simulink model "IMP_SIMPLE"  (R2022a)
settings: Solver=VariableStepAuto  StartTime=0.0  StopTime=30  RelTol=1e-3
undefined symbols (not defined in the file): Ad, Ap, Bd, Bp, Cp, ka, ki
libraries: simulink x1
settings Model: Creator=Eduardo Toro Bernal  LastModifiedBy=Eduardo Toro Bernal

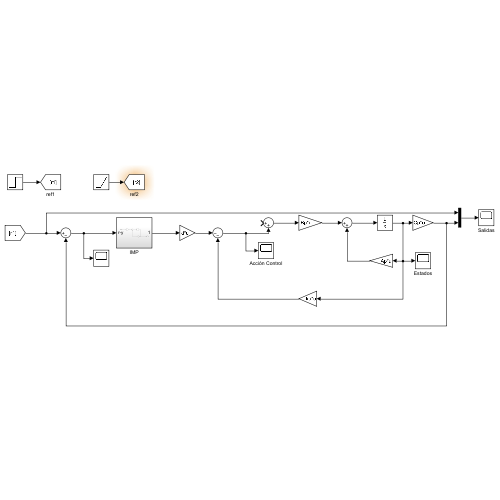
[thumbnail: Simulink's stored preview of the top-level diagram]
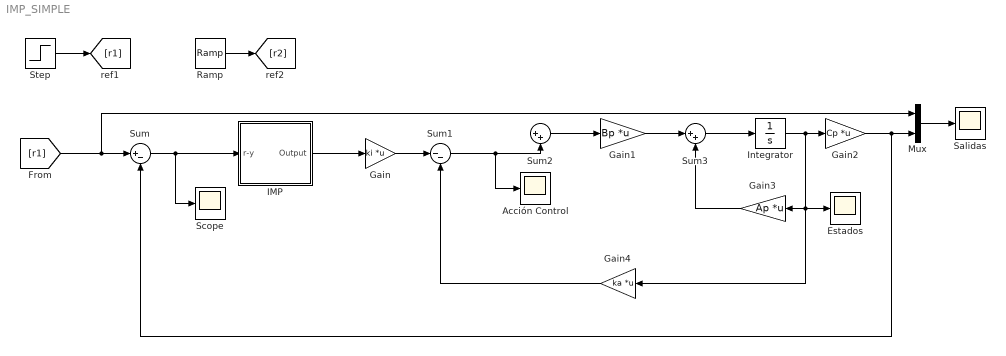
== system IMP_SIMPLE ==
  Acción Control : Scope
  Estados : Scope
  Gain : Gain  Gain=ki  Multiplication=Matrix(K*u)
  Gain1 : Gain  Gain=Bp  Multiplication=Matrix(K*u)
  Gain2 : Gain  Gain=Cp  Multiplication=Matrix(K*u)
  Gain3 : Gain  Gain=Ap  Multiplication=Matrix(K*u)
  Gain4 : Gain  Gain=ka  Multiplication=Matrix(K*u)
  IMP : Subsystem
  Integrator : Integrator
  Mux : Mux  Inputs=2
  Ramp : simulink/Sources/Ramp  slope=1  start=0  InitialOutput=0
  Salidas : Scope
  Scope : Scope
  Step : Step  SampleTime=0
  Sum : Sum  Inputs=|+-
  Sum1 : Sum  Inputs=|--
  Sum2 : Sum  Inputs=|++
  Sum3 : Sum  Inputs=|++
  wires:
  Sum/1 -> Scope/1, IMP/1(r-y)
  IMP/1(Output) -> Gain/1
  Gain/1 -> Sum1/1
  Sum1/1 -> Acción Control/1, Sum2/2
  Sum2/1 -> Gain1/1
  Gain1/1 -> Sum3/1
  Sum3/1 -> Integrator/1
  Integrator/1 -> Estados/1, Gain4/1, Gain3/1, Gain2/1
  Mux/1 -> Salidas/1
  Gain2/1 -> Sum/2, Mux/2
  [r1] -> Mux/1, Sum/1
  Gain3/1 -> Sum3/2
  Gain4/1 -> Sum1/2
  Step/1 -> [r1]
  Ramp/1 -> [r2]

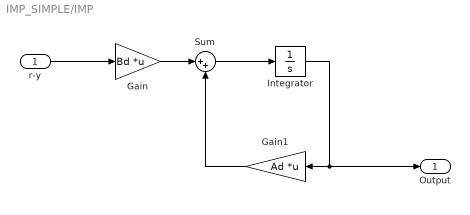
== system IMP_SIMPLE/IMP ==
  r-y : Inport
  Gain : Gain  Gain=Bd  Multiplication=Matrix(K*u)
  Gain1 : Gain  Gain=Ad  Multiplication=Matrix(K*u)
  Integrator : Integrator
  Sum : Sum  Inputs=|++
  Output : Outport
  wires:
  r-y/1 -> Gain/1
  Sum/1 -> Integrator/1
  Integrator/1 -> Output/1, Gain1/1
  Gain/1 -> Sum/1
  Gain1/1 -> Sum/2
